simulink model "SearchAreaOptimization_SensorNetwork_version_v2"  (R2019a)
settings: Solver=FixedStepAuto  StartTime=0.0  StopTime=P.Sim_Time  FixedStep=0.1  RelTol=1e-3
values from neighbouring files (symbols this model uses):
  P = cumsum(p(ant(k),:))    [Problem1_TSP_AntSystem.m]    (also in TSP_AntSystem.m)
undefined symbols (not defined in the file or in its folder): drawVehicles, GeneralSensor, SensorNetwork_Control, StateEstimator, WaypointControl
settings Model: Creator=risc_charlie  LastModifiedBy=risc_charlie

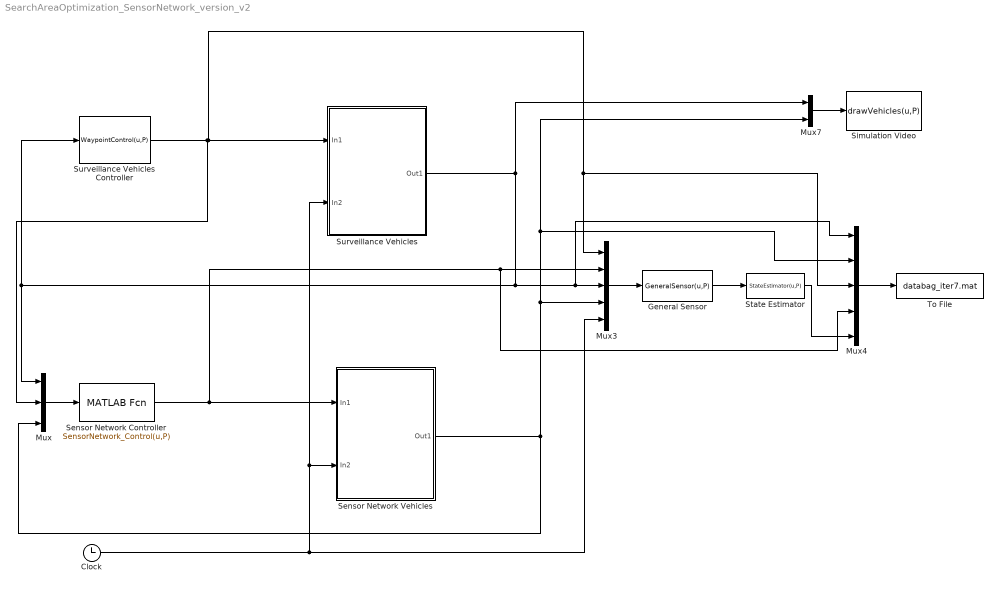
== system SearchAreaOptimization_SensorNetwork_version_v2 ==
  Clock : Clock
  General Sensor : MATLABFcn  MATLABFcn=GeneralSensor(u,P)  OutputDimensions=P.NumVeh*2+P.NumSenVeh*2+P.NumVeh*P.NumVeh+P.NumSenVeh*P.NumSenVeh+P.NumVeh*P.NumSenVeh+P.NumVeh*P.NumLm+P.NumSenVeh*P.NumLm+1
  Mux : Mux  Inputs=3
  Mux3 : Mux  Inputs=5
  Mux4 : Mux  Inputs=5
  Mux7 : Mux  Inputs=2
  Sensor Network Controller : MATLABFcn  MATLABFcn=SensorNetwork_Control(u,P)  OutputDimensions=4*2
  Sensor Network Vehicles : Subsystem
  Simulation Video : MATLABFcn  MATLABFcn=drawVehicles(u,P)  OutputDimensions=0
  State Estimator : MATLABFcn  MATLABFcn=StateEstimator(u,P)  OutputDimensions=(P.NumVeh+P.NumSenVeh)*2*3
  Surveillance Vehicles : Subsystem
  Surveillance Vehicles Controller : MATLABFcn  MATLABFcn=WaypointControl(u,P)  OutputDimensions=12
  To File : ToFile  Filename=databag_iter7.mat  MatrixName=data  SaveFormat=Timeseries
  wires:
  Surveillance Vehicles Controller/1 -> Mux/2, Surveillance Vehicles/1(In1), Mux4/3, Mux3/1
  Mux3/1 -> General Sensor/1
  General Sensor/1 -> State Estimator/1
  Mux4/1 -> To File/1
  Clock/1 -> Sensor Network Vehicles/2(In2), Surveillance Vehicles/2(In2), Mux3/5
  Surveillance Vehicles/1(Out1) -> Mux7/1, Mux3/3, Mux4/1, Mux/1, Surveillance Vehicles Controller/1
  Sensor Network Controller/1 -> Mux4/4, Mux3/2, Sensor Network Vehicles/1(In1)
  Mux7/1 -> Simulation Video/1
  Sensor Network Vehicles/1(Out1) -> Mux4/2, Mux7/2, Mux3/4, Mux/3
  State Estimator/1 -> Mux4/5
  Mux/1 -> Sensor Network Controller/1

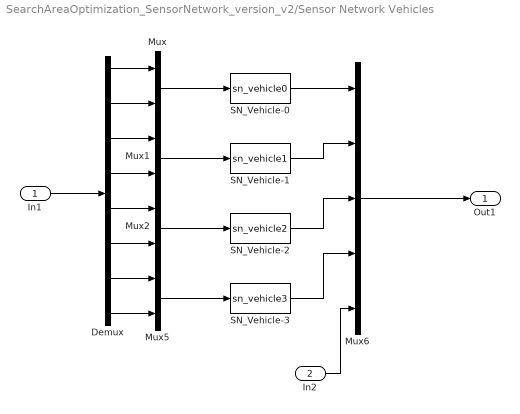
== system SearchAreaOptimization_SensorNetwork_version_v2/Sensor Network Vehicles ==
  In1 : Inport
  In2 : Inport  Port=2
  Demux : Demux  Outputs=8
  Mux{,1..2,5} (4 alike) : Mux  Inputs=2
  Mux6 : Mux  Inputs=5
  SN_Vehicle-0 : S-Function  FunctionName=sn_vehicle0  Parameters=P  SFunctionDeploymentMode=off  EnableBusSupport=off
  SN_Vehicle-1 : S-Function  FunctionName=sn_vehicle1  Parameters=P  SFunctionDeploymentMode=off  EnableBusSupport=off
  SN_Vehicle-2 : S-Function  FunctionName=sn_vehicle2  Parameters=P  SFunctionDeploymentMode=off  EnableBusSupport=off
  SN_Vehicle-3 : S-Function  FunctionName=sn_vehicle3  Parameters=P  SFunctionDeploymentMode=off  EnableBusSupport=off
  Out1 : Outport
  wires:
  Demux/2 -> Mux/2
  Demux/1 -> Mux/1
  Demux/4 -> Mux1/2
  Mux6/1 -> Out1/1
  Mux2/1 -> SN_Vehicle-2/1
  Mux/1 -> SN_Vehicle-0/1
  Demux/5 -> Mux2/1
  Demux/7 -> Mux5/1
  In2/1 -> Mux6/5
  In1/1 -> Demux/1
  Demux/8 -> Mux5/2
  SN_Vehicle-0/1 -> Mux6/1
  Demux/6 -> Mux2/2
  SN_Vehicle-2/1 -> Mux6/3
  SN_Vehicle-3/1 -> Mux6/4
  Mux1/1 -> SN_Vehicle-1/1
  SN_Vehicle-1/1 -> Mux6/2
  Mux5/1 -> SN_Vehicle-3/1
  Demux/3 -> Mux1/1

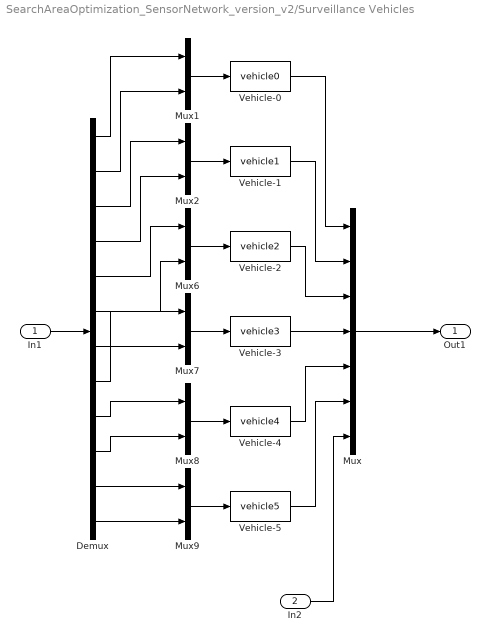
== system SearchAreaOptimization_SensorNetwork_version_v2/Surveillance Vehicles ==
  In1 : Inport
  In2 : Inport  Port=2
  Demux : Demux  Outputs=12
  Mux : Mux  Inputs=7
  Mux{1..2,6..9} (6 alike) : Mux  Inputs=2
  Vehicle-0 : S-Function  FunctionName=vehicle0  Parameters=P  SFunctionDeploymentMode=off  EnableBusSupport=off
  Vehicle-1 : S-Function  FunctionName=vehicle1  Parameters=P  SFunctionDeploymentMode=off  EnableBusSupport=off
  Vehicle-2 : S-Function  FunctionName=vehicle2  Parameters=P  SFunctionDeploymentMode=off  EnableBusSupport=off
  Vehicle-3 : S-Function  FunctionName=vehicle3  Parameters=P  SFunctionDeploymentMode=off  EnableBusSupport=off
  Vehicle-4 : S-Function  FunctionName=vehicle4  Parameters=P  SFunctionDeploymentMode=off  EnableBusSupport=off
  Vehicle-5 : S-Function  FunctionName=vehicle5  Parameters=P  SFunctionDeploymentMode=off  EnableBusSupport=off
  Out1 : Outport
  wires:
  Demux/5 -> Mux6/1
  Mux9/1 -> Vehicle-5/1
  Mux6/1 -> Vehicle-2/1
  Demux/9 -> Mux8/1
  Vehicle-0/1 -> Mux/1
  Demux/1 -> Mux1/1
  In1/1 -> Demux/1
  Demux/2 -> Mux1/2
  Vehicle-4/1 -> Mux/5
  Demux/3 -> Mux2/1
  Demux/4 -> Mux2/2
  In2/1 -> Mux/7
  Vehicle-3/1 -> Mux/4
  Mux2/1 -> Vehicle-1/1
  Demux/10 -> Mux8/2
  Mux7/1 -> Vehicle-3/1
  Demux/6 -> Mux6/2
  Mux8/1 -> Vehicle-4/1
  Vehicle-5/1 -> Mux/6
  Demux/7 -> Mux7/1
  Vehicle-1/1 -> Mux/2
  Demux/11 -> Mux9/1
  Demux/8 -> Mux7/2
  Mux1/1 -> Vehicle-0/1
  Mux/1 -> Out1/1
  Demux/12 -> Mux9/2
  Vehicle-2/1 -> Mux/3
